simulink model "MMP_simulink_example"  (R2018b)
settings: Solver=VariableStepAuto  StartTime=0.0  StopTime=t_run  RelTol=1e-3
values from neighbouring files (symbols this model uses):
  a = a(2:end)    [IIR_MMP.m]    (also in MMP.m = -1*[Apara(2:end)';zeros(L*(m-1)-m+k,1)]; a_prd.m = conv(a,[1 -2*alpha*cos(2*pi*Ts*freqinHz(i)) alpha^2]))
  Amp = [1 0.8 0.3]    [MMP_simulink.m]    (also in prediction_test.m = [1 0.8])
  B = 0    [IIR_MMP.m]    (also in lattice_filter.m = [cos(th2)*sin(th); -cos(th2)*cos(th)])
  f = [1.2 1.67 2.4]    [FIR_MMP_example.m]    (also in IIR_MMP_example.m; MMP_simulink.m; MMPexample.m; mainIIR_MMP.m = [fN*0.3,fN*0.6,fN*1.3,fN*1.6,fN*1.8,fN*0.12,fN*1.5])
  L = 4    [FIR_MMP_example.m]    (also in IIR_MMP_example.m; MMP_prediction_general.m = 6; MMP_simulink.m; MMPexample.m)
  Phi = [0.6 0.3 1.4]    [MMP_simulink.m]    (also in prediction_test.m = [0.6 0])
  Tsf = 0.1    [FIR_MMP_example.m]    (also in IIR_MMP_example.m; MMP_prediction_general.m = 0.008; MMP_simulink.m = 0.025; prediction_test.m = 0.008)
  Tss = Tsf*L    (= 0.4)    [FIR_MMP_example.m]    (also in IIR_MMP_example.m; MMP_prediction_general.m = 0.048; MMP_simulink.m = 0.1; prediction_test.m = 0.048)
  W = FIR_MMP(Apara, L, p)    [FIR_MMP_example.m]    (also in MMP.m = zeros(L-1,m); MMP_prediction_general.m = FIR_MMP(Apara, L, p, predic_step); MMP_simulink.m; MMPexample.m = MMP(Apara, L, p))
libraries: simulink x1
settings Model: Creator=macs  LastModifiedBy=macs

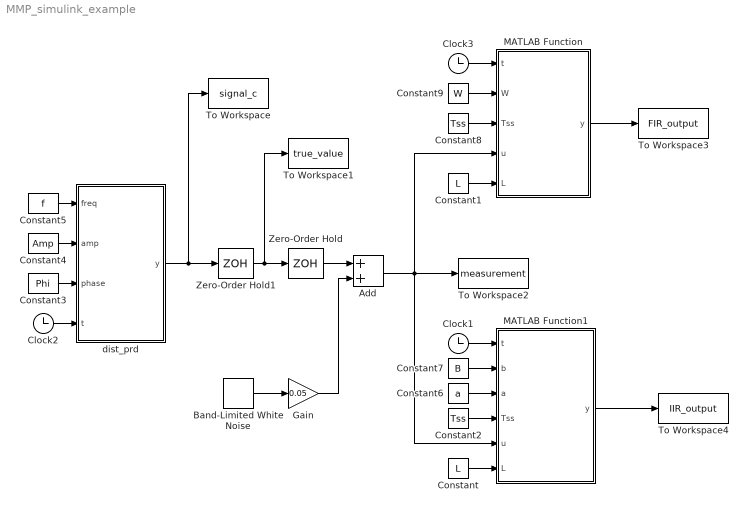
== system MMP_simulink_example ==
  " dist_prd" : MATLAB Function  TreatAsAtomicUnit=on
  Add : Sum
  Band-Limited White Noise : simulink/Sources/Band-Limited White Noise  Cov=[0.1]  Ts=Tss  seed=[23341]
  Clock1 : Clock
  Clock2 : Clock
  Clock3 : Clock
  Constant : Constant  Value=L
  Constant1 : Constant  Value=L
  Constant2 : Constant  Value=Tss
  Constant3 : Constant  Value=Phi
  Constant4 : Constant  Value=Amp
  Constant5 : Constant  Value=f
  Constant6 : Constant  Value=a
  Constant7 : Constant  Value=B
  Constant8 : Constant  Value=Tss
  Constant9 : Constant  Value=W
  Gain : Gain  Gain=0.05
  MATLAB Function : MATLAB Function  TreatAsAtomicUnit=on
  MATLAB Function1 : MATLAB Function  TreatAsAtomicUnit=on
  To Workspace : ToWorkspace  VariableName=signal_c  SaveFormat=Structure With Time  SampleTime=-1
  To Workspace1 : ToWorkspace  VariableName=true_value  SaveFormat=Structure With Time  SampleTime=-1
  To Workspace2 : ToWorkspace  VariableName=measurement  SaveFormat=Structure With Time  SampleTime=-1
  To Workspace3 : ToWorkspace  VariableName=FIR_output  SaveFormat=Structure With Time  SampleTime=-1
  To Workspace4 : ToWorkspace  VariableName=IIR_output  SaveFormat=Structure With Time  SampleTime=-1
  Zero-Order Hold : ZeroOrderHold  SampleTime=Tss
  Zero-Order Hold1 : ZeroOrderHold  SampleTime=Tsf
  wires:
  Constant3/1 -> " dist_prd"/3(phase)
  Constant4/1 -> " dist_prd"/2(amp)
  Constant5/1 -> " dist_prd"/1(freq)
  Clock2/1 -> " dist_prd"/4(t)
  Band-Limited White Noise/1 -> Gain/1
  " dist_prd"/1(y) -> To Workspace/1, Zero-Order Hold1/1
  Zero-Order Hold/1 -> Add/1
  Add/1 -> To Workspace2/1, MATLAB Function1/5(u), MATLAB Function/4(u)
  Constant/1 -> MATLAB Function1/6(L)
  Constant1/1 -> MATLAB Function/5(L)
  Constant2/1 -> MATLAB Function1/4(Tss)
  Constant6/1 -> MATLAB Function1/3(a)
  Constant7/1 -> MATLAB Function1/2(b)
  Clock1/1 -> MATLAB Function1/1(t)
  Constant8/1 -> MATLAB Function/3(Tss)
  Clock3/1 -> MATLAB Function/1(t)
  Constant9/1 -> MATLAB Function/2(W)
  Zero-Order Hold1/1 -> To Workspace1/1, Zero-Order Hold/1
  MATLAB Function/1(y) -> To Workspace3/1
  MATLAB Function1/1(y) -> To Workspace4/1
  Gain/1 -> Add/2

== matlab function MMP_simulink_example/ dist_prd ==
  settings: updateMethod=DISCRETE  sampleTime=Tsc
  data: freq input; y output; amp input; phase input; t input
function y = sig_prd(freq,amp,phase,t)
y = 0;

for i=1:length(freq)
    y = y + amp(i)*sin(2*pi*freq(i)*t+phase(i));
end

end

== matlab function MMP_simulink_example/MATLAB Function ==
  settings: updateMethod=DISCRETE  sampleTime=Tsf
  data: t input; W input; Tss input; u input; y output; L input
function y = FIR_predictor(t, W, Tss, u, L)
% Hui Xiao 10-14-2016
persistent phi;
persistent ylast;
persistent tlast;
[~,m] = size(W);
if isempty(phi)
    phi = zeros(m,1);
    tlast = t;
    ylast = 0;
end

%if this function is called at a same time multiple times,
%just update the phi table once.
if t == tlast
    y = ylast;
    return
end
tlast = t;

Tsf = Tss/L;
if (mod(t,Tss) > -Tsf/10) && (mod(t,Tss) < Tsf/10)
    %update phi
    for i=m:-1:2
        phi(i)=phi(i-1);
    end
    phi(1)=u;
    %disp(t)
    %disp(phi)
    y = u;
    ylast = y;
else
    index = round(mod(t,Tss)/Tsf);
    y = 0;
    for i = 1:m
        y=y+W(index,i)*phi(i);
        %disp(index)
    end
    ylast = y;
end
end

== matlab function MMP_simulink_example/MATLAB Function1 ==
  settings: updateMethod=DISCRETE  sampleTime=Tsf
  data: t input; b input; a input; Tss input; u input; y output; L input
function y = IIR_predictor(t, b, a, Tss, u, L)
% Hui Xiao 1-17-2017
persistent phi_d;
persistent phi_y;
persistent ylast;
persistent tlast;
[~,m] = size(b);
if isempty(phi_d)   %Initialization
    phi_d = zeros(m,1);
    phi_y = zeros(size(b)); 
    tlast = t;
    ylast = 0;
end

%if this function is called at a same time multiple times,
%just update the phi table once.
if t == tlast
    y = ylast;
    return
end
tlast = t;

Tsf = Tss/L;
if (mod(t,Tss) > -Tsf/10) && (mod(t,Tss) < Tsf/10)
    %update phi_d
    for i = m:-1:2
        phi_d(i)=phi_d(i-1);
    end
    phi_d(1)=u;
    %disp(t)
    %disp(phi)
    y = u;
    ylast = y;
else
    r = round(mod(t,Tss)/Tsf);
    y = 0;
    for i = 1:m
        y=y+b(r,i)*phi_d(i)-a(i)*phi_y(r,i);
        %disp(index)
    end
    ylast = y;
    % update phi_y
    for i = m:-1:2
        phi_y(r,i)=phi_y(r,i-1);
    end
    phi_y(r,1)=y;
end 
end
